simulink model "sampleModel1556"  (R2023a)
settings: Solver=VariableStepAuto  StartTime=0.0  StopTime=10.0  RelTol=1e-3
libraries: hdlsllib x6, simulink x1
settings Model: Creator=user1  LastModifiedBy=user1

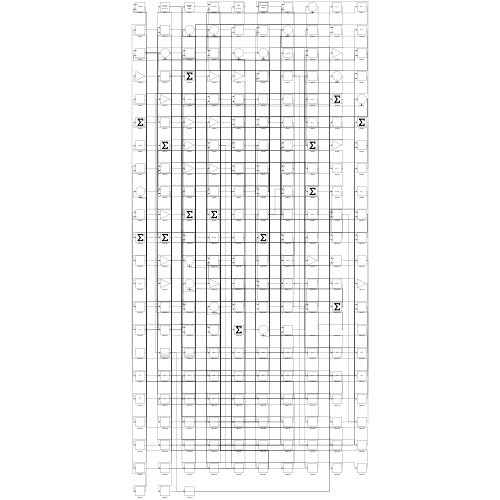
[thumbnail: Simulink's stored preview of the top-level diagram]
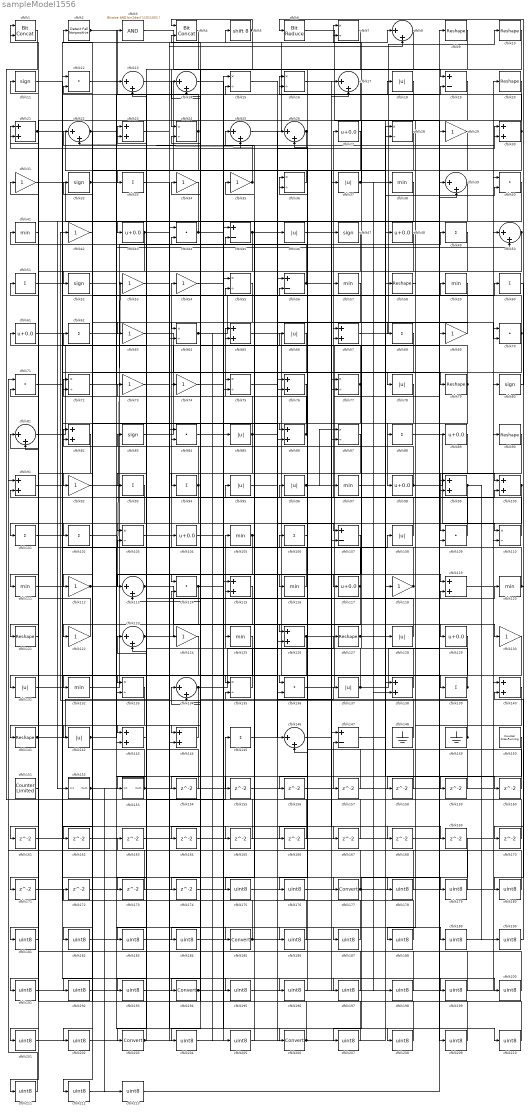
== system sampleModel1556 ==
  cfblk1 : hdlsllib/Logic and Bit Operations/Bit Concat  numInputs=2
  cfblk{9..10,20,58,79,90,121,127,141} (9 alike) : Reshape
  cfblk{21,23,30,65,67,76,82,86,91,99..100,115,119,126,138,140,143..144} (18 alike) : Sum
  cfblk{33,49,51,60,62,68,88,93..94,101..102,106,139,145} (14 alike) : Sum  Inputs=+
  cfblk{7,15..16,24,28,36,55,64,72,75,77,87,103,110,133,135} (16 alike) : Product  Inputs=*/  RndMeth=Zero  SaturateOnIntegerOverflow=on
  cfblk{27,43,48,61,89,98,104,117,129} (9 alike) : Bias  Bias=0.0  SaturateOnIntegerOverflow=off
  cfblk{38,41,57,59,97,105,111,116,120,125,132} (11 alike) : MinMax
  cfblk{19,45,56,107,147} (5 alike) : Sum  Inputs=+-
  cfblk{18,37,46,66,78,85,95..96,108,128,131,137,142} (13 alike) : Abs  SaturateOnIntegerOverflow=off
  cfblk{12,40,44,70..71,84,109,114,136} (9 alike) : DotProduct  OutDataTypeStr=Inherit: Inherit via internal rule
  cfblk{11,32,47,52,80,83} (6 alike) : Signum
  cfblk{29,31,34..35,42,53..54,63,69,73..74,92,112,118,122,124,130} (17 alike) : Gain
  cfblk{8,13..14,17,22,25..26,39,50,81,113,123,134,146} (14 alike) : Sum  Inputs=|++
  cfblk148 : Ground
  cfblk149 : Ground
  cfblk150 : hdlsllib/Sources/Counter Free-Running  NumBits=16  tsamp=-1
  cfblk151 : hdlsllib/Sources/Counter Limited  uplimit=7  tsamp=-1
  cfblk152 : Subsystem
      settings: LibrarySourceBlock=|
      | hdlsllib/Ports &
      | Subsystems/Subsystem
  cfblk153 : Subsystem
      settings: LibrarySourceBlock=|
      | hdlsllib/Ports &
      | Subsystems/Subsystem
  cfblk{154..174} (21 alike) : Delay  SampleTime=1
  cfblk{175..176,178..184,186..193,195..202,204..205,207..213} (34 alike) : DataTypeConversion  OutDataTypeStr=uint8  SaturateOnIntegerOverflow=off  RndMeth=Floor
  cfblk{177,185,194,203,206} (5 alike) : DataTypeConversion  SaturateOnIntegerOverflow=off  RndMeth=Floor
  cfblk2 : hdlsllib/Logic and Bit Operations/Detect Fall Nonpositive  vinit=0  OutDataTypeStr=boolean
  cfblk3 : simulink/Logic and Bit Operations/Bitwise Operator  logicop=AND  UseBitMask=on  BitMask=bin2dec('11011001')  BitMaskRealWorld=Stored Integer
      settings: LibrarySourceBlock=|
      | hdlsllib/Logic and Bit
      | Operations/Bitwise
      | Operator
  cfblk4 : hdlsllib/Logic and Bit Operations/Bit Concat  numInputs=2
  cfblk5 : ArithShift  BitShiftNumber=8
  cfblk6 : hdlsllib/Logic and Bit Operations/Bit Reduce  mode=AND
  wires:
  cfblk44/1 -> cfblk43/1, cfblk126/2
  cfblk149/1 -> cfblk42/1, cfblk113/2
  cfblk56/1 -> cfblk152/1(In1), cfblk169/1
  cfblk120/1 -> cfblk13/2, cfblk180/1
  cfblk65/1 -> cfblk139/1
  cfblk67/1 -> cfblk10/1
  cfblk132/1 -> cfblk49/1
  cfblk29/1 -> cfblk112/1
  cfblk1/1 -> cfblk145/1
  cfblk122/1 -> cfblk21/1
  cfblk108/1 -> cfblk27/1
  cfblk135/1 -> cfblk105/1
  cfblk152/1(Out1) -> cfblk167/1, cfblk213/1
  cfblk129/1 -> cfblk131/1
  cfblk112/1 -> cfblk53/1, cfblk187/1
  cfblk79/1 -> cfblk98/1, cfblk65/2
  cfblk24/1 -> cfblk3/1, cfblk143/2
  cfblk136/1 -> cfblk120/1
  cfblk25/1 -> cfblk7/1
  cfblk118/1 -> cfblk54/1, cfblk66/1
  cfblk45/1 -> cfblk70/2, cfblk75/2
  cfblk30/1 -> cfblk116/1, cfblk16/1, cfblk184/1
  cfblk22/1 -> cfblk52/1, cfblk208/1
  cfblk130/1 -> cfblk133/1
  cfblk68/1 -> cfblk132/1
  cfblk2/1 -> cfblk133/2, cfblk119/1
  cfblk96/1 -> cfblk36/1, cfblk9/1, cfblk48/1, cfblk87/1
  cfblk43/1 -> cfblk104/1, cfblk171/1
  cfblk36/1 -> cfblk33/1
  cfblk49/1 -> cfblk122/1
  cfblk94/1 -> cfblk102/1, cfblk23/2
  cfblk77/1 -> cfblk34/1, cfblk86/1
  cfblk125/1 -> cfblk194/1
  cfblk66/1 -> cfblk153/1(In1)
  cfblk6/1 -> cfblk118/1
  cfblk141/1 -> cfblk8/1, cfblk108/1
  cfblk116/1 -> cfblk81/1
  cfblk99/1 -> cfblk154/1, cfblk190/1
  cfblk62/1 -> cfblk177/1
  cfblk80/1 -> cfblk6/1
  cfblk101/1 -> cfblk67/1
  cfblk133/1 -> cfblk141/1
  cfblk13/1 -> cfblk146/1
  cfblk50/1 -> cfblk63/1, cfblk64/2, cfblk212/1
  cfblk100/1 -> cfblk126/1, cfblk121/1
  cfblk5/1 -> cfblk93/1, cfblk4/1
  cfblk46/1 -> cfblk47/1
  cfblk97/1 -> cfblk130/1
  cfblk37/1 -> cfblk7/2, cfblk40/2, cfblk138/2
  cfblk104/1 -> cfblk45/1
  cfblk151/1 -> cfblk1/1
  cfblk126/1 -> cfblk29/1, cfblk164/1
  cfblk109/1 -> cfblk81/2
  cfblk81/1 -> cfblk15/1
  cfblk127/1 -> cfblk160/1, cfblk198/1
  cfblk119/1 -> cfblk20/1
  cfblk41/1 -> cfblk101/1
  cfblk88/1 -> cfblk110/1
  cfblk21/1 -> cfblk58/1, cfblk79/1, cfblk16/2, cfblk86/2
  cfblk153/1(Out1) -> cfblk72/1, cfblk40/1
  cfblk110/1 -> cfblk95/1
  cfblk64/1 -> cfblk57/1, cfblk205/1
  cfblk9/1 -> cfblk146/2
  cfblk139/1 -> cfblk67/2, cfblk41/1
  cfblk145/1 -> cfblk137/1
  cfblk15/1 -> cfblk56/1
  cfblk69/1 -> cfblk68/1
  cfblk55/1 -> cfblk144/1
  cfblk89/1 -> cfblk114/1
  cfblk134/1 -> cfblk127/1, cfblk193/1
  cfblk8/1 -> cfblk64/1
  cfblk34/1 -> cfblk103/1
  cfblk85/1 -> cfblk73/1, cfblk144/2, cfblk30/2
  cfblk83/1 -> cfblk37/1
  cfblk14/1 -> cfblk206/1
  cfblk59/1 -> cfblk94/1
  cfblk98/1 -> cfblk100/1, cfblk75/1, cfblk4/2
  cfblk144/1 -> cfblk142/1
  cfblk92/1 -> cfblk100/2
  cfblk117/1 -> cfblk36/2, cfblk134/2
  cfblk32/1 -> cfblk50/2, cfblk78/1
  cfblk90/1 -> cfblk109/1
  cfblk51/1 -> cfblk5/1
  cfblk4/1 -> cfblk24/1
  cfblk105/1 -> cfblk35/1, cfblk204/1
  cfblk78/1 -> cfblk113/1
  cfblk138/1 -> cfblk82/1
  cfblk114/1 -> cfblk30/1, cfblk192/1
  cfblk128/1 -> cfblk61/1
  cfblk28/1 -> cfblk77/2
  cfblk106/1 -> cfblk26/2
  cfblk111/1 -> cfblk135/1
  cfblk70/1 -> cfblk2/1, cfblk87/2
  cfblk95/1 -> cfblk107/1
  cfblk58/1 -> cfblk88/1
  cfblk113/1 -> cfblk129/1, cfblk119/2
  cfblk61/1 -> cfblk59/1
  cfblk143/1 -> cfblk23/1
  cfblk148/1 -> cfblk56/2
  cfblk63/1 -> cfblk128/1
  cfblk142/1 -> cfblk106/1, cfblk155/1
  cfblk48/1 -> cfblk92/1
  cfblk123/1 -> cfblk99/1, cfblk13/1, cfblk143/1
  cfblk16/1 -> cfblk109/2
  cfblk72/1 -> cfblk18/1
  cfblk11/1 -> cfblk82/2
  cfblk121/1 -> cfblk51/1
  cfblk3/1 -> cfblk19/1
  cfblk93/1 -> cfblk111/1
  cfblk27/1 -> cfblk136/1
  cfblk147/1 -> cfblk28/1
  cfblk18/1 -> cfblk117/1
  cfblk115/1 -> cfblk203/1
  cfblk26/1 -> cfblk25/2, cfblk156/1
  cfblk35/1 -> cfblk22/1, cfblk22/2
  cfblk107/1 -> cfblk123/2
  cfblk146/1 -> cfblk19/2
  cfblk75/1 -> cfblk60/1
  cfblk54/1 -> cfblk136/2
  cfblk23/1 -> cfblk8/2
  cfblk137/1 -> cfblk69/1, cfblk25/1
  cfblk73/1 -> cfblk15/2
  cfblk86/1 -> cfblk65/1, cfblk24/2
  cfblk12/1 -> cfblk185/1
  cfblk154/1 -> cfblk123/1
  cfblk155/1 -> cfblk147/2
  cfblk156/1 -> cfblk28/2
  cfblk157/1 -> cfblk55/2
  cfblk19/1 -> cfblk158/1
  cfblk158/1 -> cfblk21/2
  cfblk33/1 -> cfblk159/1
  cfblk159/1 -> cfblk72/2
  cfblk160/1 -> cfblk77/1
  cfblk40/1 -> cfblk161/1
  cfblk161/1 -> cfblk50/1
  cfblk57/1 -> cfblk162/1
  cfblk163/1 -> cfblk99/2
  cfblk52/1 -> cfblk165/1
  cfblk165/1 -> cfblk103/2
  cfblk20/1 -> cfblk166/1
  cfblk166/1 -> cfblk135/2
  cfblk167/1 -> cfblk134/1
  cfblk71/1 -> cfblk168/1
  cfblk168/1 -> cfblk70/1
  cfblk60/1 -> cfblk170/1
  cfblk170/1 -> cfblk45/2
  cfblk171/1 -> cfblk110/2
  cfblk172/1 -> cfblk107/2
  cfblk10/1 -> cfblk173/1
  cfblk173/1 -> cfblk1/2
  cfblk47/1 -> cfblk174/1
  cfblk174/1 -> cfblk46/1
  cfblk38/1 -> cfblk175/1
  cfblk175/1 -> cfblk89/1
  cfblk87/1 -> cfblk176/1
  cfblk176/1 -> cfblk38/1
  cfblk177/1 -> cfblk71/2, cfblk44/1
  cfblk150/1 -> cfblk178/1
  cfblk178/1 -> cfblk62/1
  cfblk91/1 -> cfblk179/1
  cfblk179/1 -> cfblk55/1
  cfblk180/1 -> cfblk91/1
  cfblk82/1 -> cfblk181/1
  cfblk181/1 -> cfblk91/2
  cfblk76/1 -> cfblk182/1
  cfblk182/1 -> cfblk157/1
  cfblk7/1 -> cfblk183/1
  cfblk183/1 -> cfblk76/1
  cfblk184/1 -> cfblk76/2
  cfblk185/1 -> cfblk97/1, cfblk83/1
  cfblk53/1 -> cfblk186/1
  cfblk186/1 -> cfblk12/1
  cfblk187/1 -> cfblk12/2
  cfblk140/1 -> cfblk188/1
  cfblk188/1 -> cfblk147/1
  cfblk164/1 -> cfblk189/1
  cfblk189/1 -> cfblk140/1
  cfblk190/1 -> cfblk140/2
  cfblk17/1 -> cfblk191/1
  cfblk191/1 -> cfblk85/1
  cfblk192/1 -> cfblk17/1
  cfblk193/1 -> cfblk17/2
  cfblk194/1 -> cfblk90/1, cfblk80/1
  cfblk102/1 -> cfblk195/1
  cfblk195/1 -> cfblk125/1
  cfblk84/1 -> cfblk196/1
  cfblk196/1 -> cfblk96/1
  cfblk162/1 -> cfblk197/1
  cfblk197/1 -> cfblk84/1
  cfblk198/1 -> cfblk84/2
  cfblk74/1 -> cfblk199/1
  cfblk199/1 -> cfblk11/1
  cfblk131/1 -> cfblk200/1
  cfblk200/1 -> cfblk74/1
  cfblk124/1 -> cfblk201/1
  cfblk201/1 -> cfblk26/1
  cfblk42/1 -> cfblk202/1
  cfblk202/1 -> cfblk124/1
  cfblk203/1 -> cfblk163/1, cfblk138/1
  cfblk204/1 -> cfblk115/1
  cfblk205/1 -> cfblk115/2
  cfblk206/1 -> cfblk172/1, cfblk114/2, cfblk44/2
  cfblk169/1 -> cfblk207/1
  cfblk207/1 -> cfblk14/1
  cfblk208/1 -> cfblk14/2
  cfblk31/1 -> cfblk209/1
  cfblk209/1 -> cfblk32/1
  cfblk103/1 -> cfblk210/1
  cfblk210/1 -> cfblk31/1
  cfblk39/1 -> cfblk211/1
  cfblk211/1 -> cfblk71/1
  cfblk212/1 -> cfblk39/1
  cfblk213/1 -> cfblk39/2

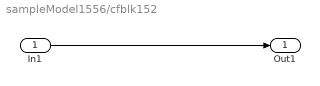
== system sampleModel1556/cfblk152 ==
  In1 : Inport
  Out1 : Outport
  wires:
  In1/1 -> Out1/1

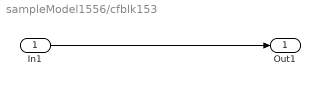
== system sampleModel1556/cfblk153 ==
  In1 : Inport
  Out1 : Outport
  wires:
  In1/1 -> Out1/1
